simulink model "single_upsample_and_mix"  (R2022a)
settings: Solver=VariableStepAuto  StartTime=0.0  StopTime=33E-5  RelTol=1e-3
PreLoadFcn:
  | Fpass = 0.029;  % Passband Frequency
  | Fstop = 0.06;   % Stopband Frequency
  | Apass = 0.01;   % Passband Ripple (dB)
  | Astop = 100;    % Stopband Attenuation (dB)
  | h = fdesign.interpolator(16, 'Lowpass', 'fp,fst,ap,ast', Fpass, Fstop, ...
  |     Apass, Astop);
  | Hd = design(h, 'equiripple', ...
  |     'MinOrder', 'any', ...
  |     'StopbandShape', 'flat', ...
  |     'SystemObject', true);
  | set(Hd, ...
  |     'CoefficientsDataType', 'Custom', ...
  |     'CustomCoefficientsDataType', numerictype([],27,26));
  | h324=Hd.Numerator();
InitFcn:
  | Fbits=32; %frequency resolution
  | Abits=16; %Sin/COS table depth is 2^Abits
  | Dbits=16; %Sin/COS table width is 1..-Dbits
  | 
  | 
  | clk = 500e+6; % Hz
  | sample_rate = 1/2e+9; % 2GHz
  | SSR = 4;%ceil((1/sample_rate)*(1/clk));
  | Tclk = 1/clk;
  | Ts = sample_rate;
  | 
  | Is = 125e6;
  | Tis = 1/Is;
  | 
  | % FIR filter chain variables
  | pos = 1000/16*[0:16]*1E6;
  | channels = [pos,fliplr(pos(2:16)).*-1];
  | 
  | Fpass = 0.029;  % Passband Frequency
  | Fstop = 0.06;   % Stopband Frequency
  | Apass = 0.01;   % Passband Ripple (dB)
  | Astop = 100;    % Stopband Attenuation (dB)
  | h = fdesign.interpolator(16, 'Lowpass', 'fp,fst,ap,ast', Fpass, Fstop, ...
  |     Apass, Astop);
  | Hd = design(h, 'equiripple', ...
  |     'MinOrder', 'any', ...
  |     'StopbandShape', 'flat', ...
  |     'SystemObject', true);
  | set(Hd, ...
  |     'CoefficientsDataType', 'Custom', ...
  |     'CustomCoefficientsDataType', numerictype([],27,26));
  | h324=Hd.Numerator();
StartFcn:
  | start_time = tic;
StopFcn:
  | stop_time = toc(start_time)/60
undefined symbols (not defined in the file or in its folder): S, vsva2197, xcvc1902
libraries: hdlBasic x32, hdlSSR x15, hdlDSPIP x4, hdlUtilities x2, dspsigattribs x1, dspmlti4 x1, dspsrcs4 x1, vmcUtilities x1
settings Model: Creator=admin  LastModifiedBy=amd
settings SolverCC: AlgebraicLoopSolver=TrustRegion
settings DataIOCC: ReturnWorkspaceOutputs=off
settings DebuggingCC: UnconnectedInputMsg=warning  UnconnectedOutputMsg=warning  UnconnectedLineMsg=warning  SFMachineParentedDataDiag=warning  ArithmeticOperatorsInVariantConditions=warning
settings SFSimCC: SimUseLocalCustomCode=off  CustomCodeUndefinedFunction=UseInterfaceOnly
settings RTWCC: RTWUseLocalCustomCode=off  DLArmComputeVersion=19.05
settings CodeAppCC: StateflowObjectComments=on

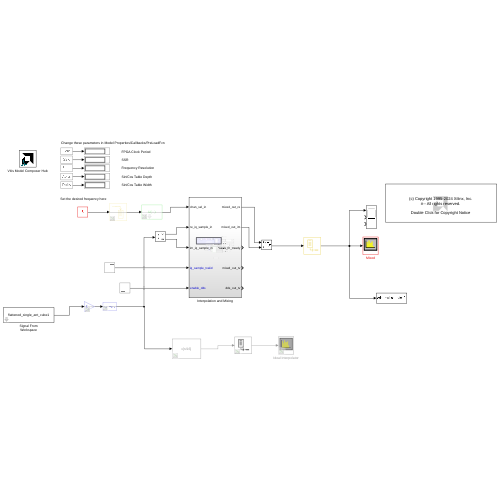
[thumbnail: Simulink's stored preview of the top-level diagram]
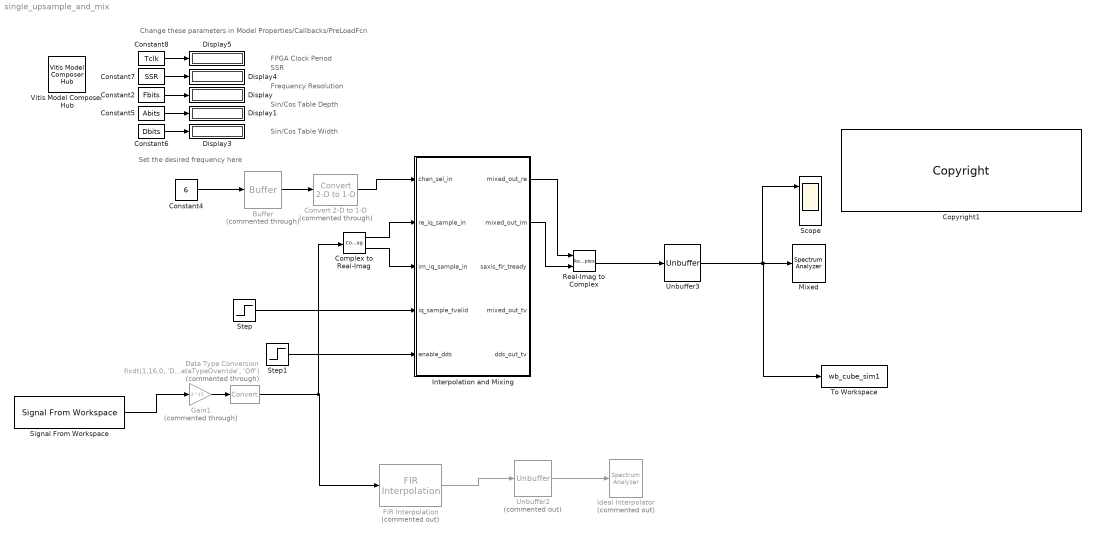
== system single_upsample_and_mix ==
  note: Frequency Resolution
  note: Set the desired frequency here
  note: Change these parameters in Model Properties/Callbacks/PreLoadFcn
  note: SSR
  note: FPGA Clock Period
  note: Sin/Cos Table Width
  note: Sin/Cos Table Depth
  Buffer : Buffer  Commented=through  N=SSR  OutputFrames=off
  Complex to Real-Imag : ComplexToRealImag
  Constant2 : Constant  Value=Fbits  OutDataTypeStr=int32  SampleTime=-1
  Constant4 : Constant  Value=6  OutDataTypeStr=fixdt(0,5,0)  SampleTime=-1
  Constant5 : Constant  Value=Abits  OutDataTypeStr=int32  SampleTime=-1
  Constant6 : Constant  Value=Dbits  OutDataTypeStr=int32  SampleTime=-1
  Constant7 : Constant  Value=SSR  OutDataTypeStr=int32  SampleTime=-1
  Constant8 : Constant  Value=Tclk  OutDataTypeStr=double  SampleTime=-1
  Convert 2-D to 1-D : dspsigattribs/Convert 2-D to 1-D  Commented=through
      settings: SourceProductBaseCode=DS
  Copyright1 : hdlUtilities/Copyright  copyrighttext="Copyright (c) 2024  by  Xilinx, Inc. All rights reserved.<br><br>This file contains proprietary, confidential information of Xilinx, Inc., is distributed under license from Xilinx, Inc., and may be used, copied and/or disclosed only pursuant to the terms of a valid license agreement with Xilinx, Inc. Xilinx hereby grants you a license to use this file solely for design, simulation, implementation and creation of design files limited to Xilinx devices or technologies. Use with non-Xilinx devices or technologies is expressly prohibited and immediately terminates your license unless covered by a separate agreement.<br><br>Xilinx is providing this design, code, or information \"as-is\" solely for use in developing programs and solutions for Xilinx devices, with no obligation on the part of Xilinx to provide support. By providing this design, code, or information as one possible implementation of this feature, application or standard, Xilinx is making no representation that this implementation is free from any claims of infringement. You are responsible for obtaining any rights you may require for your implementation. Xilinx expressly disclaims any warranty whatsoever with respect to the adequacy of the implementation, including but not limited to any warranties or representations that this implementation is free from claims of infringement, implied warranties of merchantability or fitness for a particular purpose.<br><br>Xilinx products are not intended for use in life support appliances, devices, or systems. Use in such applications is expressly prohibited.<br><br>Any modifications that are made to the Source Code are done at the user's sole risk and will be unsupported.<br><br>This copyright and support notice must be retained as part of this text at all times. (c) Copyright 1995-2024 Xilinx, Inc. All rights reserved."  block_type=copyright
  Data Type Conversion : DataTypeConversion  Commented=through  OutDataTypeStr=fixdt(1,16,0, 'DataTypeOverride', 'Off')  SaturateOnIntegerOverflow=off  RndMeth=Floor  LockScale=on
  Display{,1,3..5} (5 alike) : Display
  FIR Interpolation : dspmlti4/FIR Interpolation  Commented=on  FilterSource=Dialog parameters  PrivateCoeffs=0  h=h512  L=16  FilterObject=FINTERP  InputProcessing=Columns as channels (frame based)  framing=Enforce single-rate processing  outputBufInitCond=0  roundingMode=Floor  overflowMode=off  firstCoeffDataTypeStr=Inherit: Same word length as input  firstCoeffMin=[]  firstCoeffMax=[]  firstCoeffLastDataTypeStr=Inherit: Same word length as input  outputDataTypeStr=Inherit: Same as accumulator  outputMin=[]  outputMax=[]  outputLastDataTypeStr=Inherit: Same as accumulator
  Gain1 : Gain  Commented=through  Gain=2^15
  Ideal Interpolator : SpectrumAnalyzer  Commented=on
  Interpolation and Mixing : Subsystem
  Mixed : SpectrumAnalyzer
  Real-Imag to Complex : RealImagToComplex
  Scope : Scope  NumInputPorts=3
  Signal From Workspace : dspsrcs4/Signal From Workspace  X=flattened_single_ant_cube1  Ts=Tis  nsamps=1  OutputAfterFinalValue=Cyclic repetition  ignoreOrWarnInputAndFrameLengths=off  OutputFrames=off
  Step : Step  Time=Tis  OutDataTypeStr=Inherit: Inherit via back propagation  SampleTime=0
  Step1 : Step  Time=Tis  OutDataTypeStr=Inherit: Inherit via back propagation  SampleTime=0
  To Workspace : ToWorkspace  VariableName=wb_cube_sim1  SaveFormat=Timeseries  SampleTime=-1
  Unbuffer2 : Unbuffer  Commented=on
  Unbuffer3 : Unbuffer
  Vitis Model Composer Hub : vmcUtilities/Vitis Model Composer Hub  Tag=genX  CodeGeneration=off  TargetDirectory=./code  ExportType=System Generator  IpVendor=xilinx.com  IpLibrary=hls  IpVersion=1.0  IpHWLanguage=Verilog  AieCompilerOptions={}  AieSimulatorOptions={}  CreateTestbench=off  TestbenchStackSize=10  RunRtlSim=off  RunCSim=off  RunAieSim=off  AieSimTimeout=50000  RunAieSimProfiling=off  LaunchVitisAnalyzer=off  PlotOutput=off  RunX86Sim=off  X86SimTimeout=10  GenHwImage=off  GenLibadfXo=off  PlatformType=Not Specified  HwSystemType=Baremetal  HwValidationTarget=hw  ProjDevice=Versal VCK190 Evaluation Platform (xcvc1902-vsva2197-2MP-e-S)  ProjDevicePart=xcvc1902-vsva2197-2MP-e-S  AIEType=AIE  SamplePeriod=-1  ClockFrequency=200  DataPathParallelism=1  xilinxfamily=versalaicore  part=xcvc1902  speed=-2MP-e-S  package=vsva2197  directory=C:/work/tmp/v7_rc2  testbench=off  incr_netlist=off  synthesis_tool=Vivado  clock_wrapper=Clock Enables  dbl_ovrd=According to Block Masks  dcm_input_clock_period=10  sysclk_period=(1e+9)/clk  simulink_period=1/clk  eval_field=0  IPInfoJsonString="{\"HDLSubsystem\":{\"SubsystemName\":\"Interpolation and Mixing\",\"IPName\":\"stap_upsampler\",\"IPLibrary\":\"VMC\",\"IPVendor\":\"User Company\",\"IPVersion\":\"1.0\"}}"  LogFileName=''  NThreads=4
  wires:
  Constant4/1 -> Buffer/1
  Buffer/1 -> Convert 2-D to 1-D/1
  Constant2/1 -> Display/1
  Constant6/1 -> Display3/1
  Constant7/1 -> Display4/1
  Constant8/1 -> Display5/1
  Unbuffer3/1 -> To Workspace/1, Mixed/1, Scope/1
  Constant5/1 -> Display1/1
  Convert 2-D to 1-D/1 -> Interpolation and Mixing/1(chan_sel_in)
  FIR Interpolation/1 -> Unbuffer2/1
  Unbuffer2/1 -> Ideal Interpolator/1
  Gain1/1 -> Data Type Conversion/1
  Signal From Workspace/1 -> Gain1/1
  Data Type Conversion/1 -> Complex to Real-Imag/1, FIR Interpolation/1
  Interpolation and Mixing/2(mixed_out_im) -> Real-Imag to Complex/2
  Interpolation and Mixing/1(mixed_out_re) -> Real-Imag to Complex/1
  Real-Imag to Complex/1 -> Unbuffer3/1
  Complex to Real-Imag/1 -> Interpolation and Mixing/2(re_iq_sample_in)
  Complex to Real-Imag/2 -> Interpolation and Mixing/3(im_iq_sample_in)
  Step/1 -> Interpolation and Mixing/4(iq_sample_tvalid)
  Step1/1 -> Interpolation and Mixing/5(enable_dds)

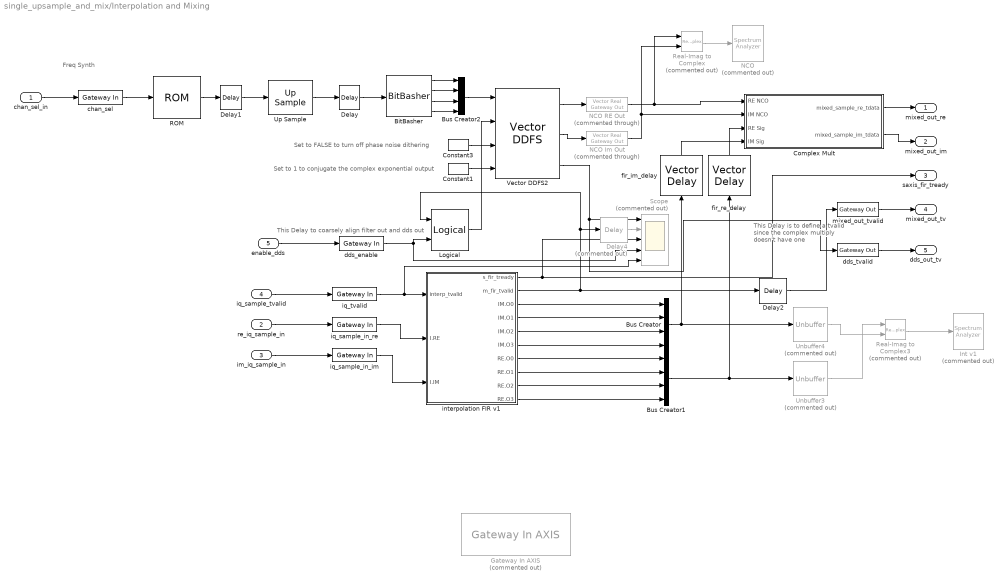
== system single_upsample_and_mix/Interpolation and Mixing ==
  note: Freq Synth
  note: Set to 1 to conjugate the complex exponential output
  note: Set to FALSE to turn off phase noise dithering
  note: This Delay to coarsely align filter out and dds out
  note: This Delay is to define a tvalid since
      | the complex multiply doesn't have one
  chan_sel_in : Inport  SampleTime=Tis
  re_iq_sample_in : Inport  Port=2
  im_iq_sample_in : Inport  Port=3
  iq_sample_tvalid : Inport  Port=4  SampleTime=Tis
  enable_dds : Inport  Port=5  SampleTime=Tclk
  BitBasher : hdlBasic/BitBasher  bitexpr=|  display_expr=off  sr_1=a  arith_type1="Signed  (2's comp)"  bin_pt1=0  sr_2=b  arith_type2="Signed  (2's comp)"  bin_pt2=0  sr_3=c  arith_type3="Signed  (2's comp)"  bin_pt3=0  sr_4=d  arith_type4="Signed  (2's comp)"  bin_pt4=0  XmcBlockStatus=1  maskContainerNames=group1  block_type=bitbasher  block_config=sysgen:BitBasher_config
      | a={e}
      | b={e}
      | c={e}
      | d={e}
  Bus Creator : BusCreator  Inputs=4
  Bus Creator1 : BusCreator  Inputs=4
  Bus Creator2 : BusCreator  Inputs=4
  Complex Mult : Subsystem
  Constant1 : hdlBasic/Constant  const=1  gui_display_data_type=Fixed-point  arith_type=Unsigned  n_bits=1  bin_pt=0  preci_type=Single  exp_width=8  frac_width=24  explicit_period=on  period=Tclk  XmcBlockStatus=1  maskContainerNames=tabcontainer1  block_type=constant  block_config=sysgen:Constant_config
  Constant3 : hdlBasic/Constant  const=1  gui_display_data_type=Boolean  arith_type=Boolean  n_bits=1  bin_pt=0  preci_type=Single  exp_width=8  frac_width=24  explicit_period=on  period=Tclk  XmcBlockStatus=1  maskContainerNames=tabcontainer1  block_type=constant  block_config=sysgen:Constant_config
  Delay : hdlBasic/Delay  rst=off  en=off  latency=1  reg_retiming=off  XmcBlockStatus=1  maskContainerNames=group1  block_type=delay  block_config=sysgen:Delay_config
  Delay1 : hdlBasic/Delay  rst=off  en=off  latency=1  reg_retiming=off  XmcBlockStatus=1  maskContainerNames=group1  block_type=delay  block_config=sysgen:Delay_config
  Delay2 : hdlBasic/Delay  rst=off  en=off  latency=5  reg_retiming=off  XmcBlockStatus=1  maskContainerNames=group1  block_type=delay  block_config=sysgen:Delay_config
  Delay4 : hdlBasic/Delay  Commented=on  rst=off  en=off  latency=13  reg_retiming=off  XmcBlockStatus=1  maskContainerNames=group1  block_type=delay  block_config=sysgen:Delay_config
  Gateway In AXIS : hdlUtilities/Gateway In AXIS  Commented=on  gui_display_data_type=Fixed-point  arith_type=Signed (2's comp)  n_bits=1  bin_pt=0  preci_type=Custom  exp_width=16  frac_width=24  quantization=Truncate  overflow=Flag as error  OutSampleTime=1  block_type=gatewayinaxi  XmcBlockStatus=1
  Int v1 : SpectrumAnalyzer  Commented=on
  Logical : hdlBasic/Logical  logical_function=OR  inputs=2  en=off  latency=1  precision=User Defined  arith_type=Boolean  n_bits=1  bin_pt=0  align_bp=on  overflow=[]  quantization=[]  XmcBlockStatus=1  maskContainerNames=tabcontainer1  block_type=logical  block_config=sysgen:Logical_config
  NCO : SpectrumAnalyzer  Commented=on
  NCO Im Out : hdlSSR/Vector Real Gateway Out  Commented=through  inherit_from_input=off  hdl_port=off  sg_ssr=4  rows=1  columns=1  UseAsDAC=off  DACChannel='1'  interface=None  automatic_assignment=on  address_offset=hex2dec('00')  intf_name=''  intf_description=''  timing_constraint=None  locs_specified=off  LOCs={}  io_standard={}  block_type=realgatewayout_ssr  XmcBlockStatus=1  sg_ssr_prev=4  maskContainerNames=group4  block_width_w=590  block_height_w=620  block_width=620  block_height=750
  NCO RE Out : hdlSSR/Vector Real Gateway Out  Commented=through  inherit_from_input=off  hdl_port=off  sg_ssr=4  rows=1  columns=1  UseAsDAC=off  DACChannel='1'  interface=None  automatic_assignment=on  address_offset=hex2dec('00')  intf_name=''  intf_description=''  timing_constraint=None  locs_specified=off  LOCs={}  io_standard={}  block_type=realgatewayout_ssr  XmcBlockStatus=1  sg_ssr_prev=4  maskContainerNames=group4  block_width_w=590  block_height_w=620  block_width=620  block_height=750
  ROM : hdlBasic/ROM  depth=32  initVector=channels*Ts*2^Fbits  distributed_mem=Distributed memory  rst=off  init_reg=0  en=off  latency=1  gui_display_data_type=Fixed-point  arith_type="Signed  (2's comp)"  n_bits=32  bin_pt=0  preci_type=Single  exp_width=8  frac_width=24  optimize=Area  use_rpm=on  simulation_type=fast_sim  XmcBlockStatus=1  maskContainerNames=tabcontainer1  block_type=sprom  block_config=sysgen:SPROM_config
  Real-Imag to Complex : RealImagToComplex  Commented=on
  Real-Imag to Complex3 : RealImagToComplex  Commented=on
  Scope : Scope  Commented=on  NumInputPorts=5
  Unbuffer3 : Unbuffer  Commented=on
  Unbuffer4 : Unbuffer  Commented=on
  Up Sample : hdlBasic/Up Sample  sample_ratio=4  copy_samples=on  en=off  latency=1  XmcBlockStatus=1  maskContainerNames=group1  block_type=usamp  block_config=sysgen:Upsample_config
  Vector DDFS2 : hdlSSR/Vector DDFS  sg_ssr=SSR  Fbits=Fbits  Abits=Abits  Dbits=Dbits  block_type=ddfs_ssr  XmcBlockStatus=1  sg_ssr_prev=4  maskContainerNames=group1
      settings: SourceProductName=Xilinx SSR Blockset
  chan_sel : hdlBasic/Gateway In  gui_display_data_type=Fixed-point  arith_type=Unsigned  n_bits=5  bin_pt=0  preci_type=Single  exp_width=8  frac_width=24  rows=1  columns=1  quantization=Truncate  overflow=Wrap  period=Tis  UseAsADC=off  ADCChannel='1'  interface=None  automatic_assignment=on  address_offset=hex2dec('00')  intf_name='channel_sel'  intf_description='0:31 mix channel select'  default_value=0  timing_constraint=None  locs_specified=off  LOCs={}  io_standard={}  inherit_from_input=off  hdl_port=on  XmcBlockStatus=1  maskContainerNames=group4  block_type=gatewayin  block_config=sysgen:gateway_in_config  block_width_w=590  block_height_w=620  block_width=640  block_height=850
  dds_enable : hdlBasic/Gateway In  gui_display_data_type=Boolean  arith_type=Boolean  n_bits=16  bin_pt=14  preci_type=Single  exp_width=8  frac_width=24  rows=1  columns=1  quantization="Round  (unbiased: +/- Inf)"  overflow=Saturate  period=Tclk  UseAsADC=off  ADCChannel='1'  interface=None  automatic_assignment=on  address_offset=hex2dec('00')  intf_name=''  intf_description=''  default_value=0  timing_constraint=None  locs_specified=off  LOCs={}  io_standard={}  inherit_from_input=off  hdl_port=on  XmcBlockStatus=1  maskContainerNames=group4  block_type=gatewayin  block_config=sysgen:gateway_in_config  block_width_w=590  block_height_w=620  block_width=640  block_height=850
  dds_tvalid : hdlBasic/Gateway Out  inherit_from_input=on  hdl_port=on  rows=1  columns=1  UseAsDAC=off  DACChannel='1'  interface=None  automatic_assignment=on  address_offset=hex2dec('00')  intf_name=''  intf_description=''  timing_constraint=None  locs_specified=off  LOCs={}  io_standard={}  XmcBlockStatus=1  maskContainerNames=group4  block_type=gatewayout  block_config=sysgen:gateway_out_config  block_width_w=590  block_height_w=620  block_width=620  block_height=750
  fir_im_delay : hdlSSR/Vector Delay  rst=off  en=off  vectorize_en=off  sg_latency=1  sg_ssr=4  reg_retiming=off  block_type=delay_ssr  XmcBlockStatus=1  sg_ssr_prev=4  maskContainerNames=group1
  fir_re_delay : hdlSSR/Vector Delay  rst=off  en=off  vectorize_en=off  sg_latency=1  sg_ssr=4  reg_retiming=off  block_type=delay_ssr  XmcBlockStatus=1  sg_ssr_prev=4  maskContainerNames=group1
  interpolation FIR v1 : Subsystem
  iq_sample_in_im : hdlBasic/Gateway In  gui_display_data_type=Fixed-point  arith_type=Signed (2's comp)  n_bits=16  bin_pt=15  preci_type=Single  exp_width=8  frac_width=24  rows=1  columns=1  quantization=Truncate  overflow=Saturate  period=Tis  UseAsADC=off  ADCChannel='1'  interface=None  automatic_assignment=on  address_offset=hex2dec('00')  intf_name=''  intf_description=''  default_value=0  timing_constraint=None  locs_specified=off  LOCs={}  io_standard={}  inherit_from_input=off  hdl_port=on  XmcBlockStatus=1  maskContainerNames=group4  block_type=gatewayin  block_config=sysgen:gateway_in_config  block_width_w=590  block_height_w=620  block_width=640  block_height=850
  iq_sample_in_re : hdlBasic/Gateway In  gui_display_data_type=Fixed-point  arith_type=Signed (2's comp)  n_bits=16  bin_pt=15  preci_type=Single  exp_width=8  frac_width=24  rows=1  columns=1  quantization=Truncate  overflow=Saturate  period=Tis  UseAsADC=off  ADCChannel='1'  interface=None  automatic_assignment=on  address_offset=hex2dec('00')  intf_name=''  intf_description=''  default_value=0  timing_constraint=None  locs_specified=off  LOCs={}  io_standard={}  inherit_from_input=off  hdl_port=on  XmcBlockStatus=1  maskContainerNames=group4  block_type=gatewayin  block_config=sysgen:gateway_in_config  block_width_w=590  block_height_w=620  block_width=640  block_height=850
  iq_tvalid : hdlBasic/Gateway In  gui_display_data_type=Boolean  arith_type=Boolean  n_bits=16  bin_pt=14  preci_type=Single  exp_width=8  frac_width=24  rows=1  columns=1  quantization="Round  (unbiased: +/- Inf)"  overflow=Saturate  period=Tis  UseAsADC=off  ADCChannel='1'  interface=None  automatic_assignment=on  address_offset=hex2dec('00')  intf_name=''  intf_description=''  default_value=0  timing_constraint=None  locs_specified=off  LOCs={}  io_standard={}  inherit_from_input=off  hdl_port=on  XmcBlockStatus=1  maskContainerNames=group4  block_type=gatewayin  block_config=sysgen:gateway_in_config  block_width_w=590  block_height_w=620  block_width=640  block_height=850
  mixed_out_tvalid : hdlBasic/Gateway Out  inherit_from_input=on  hdl_port=on  rows=1  columns=1  UseAsDAC=off  DACChannel='1'  interface=None  automatic_assignment=on  address_offset=hex2dec('00')  intf_name=''  intf_description=''  timing_constraint=None  locs_specified=off  LOCs={}  io_standard={}  XmcBlockStatus=1  maskContainerNames=group4  block_type=gatewayout  block_config=sysgen:gateway_out_config  block_width_w=590  block_height_w=620  block_width=620  block_height=750
  mixed_out_re : Outport  SampleTime=Tclk
  mixed_out_im : Outport  Port=2  SampleTime=Tclk
  saxis_fir_tready : Outport  Port=3  SampleTime=Tclk
  mixed_out_tv : Outport  Port=4  SampleTime=Tclk
  dds_out_tv : Outport  Port=5  SampleTime=Tclk
  wires:
  BitBasher/1 -> Bus Creator2/1
  iq_sample_tvalid/1 -> iq_tvalid/1
  iq_tvalid/1 -> Scope/5, interpolation FIR v1/1("interp_tvalid ")
  iq_sample_in_im/1 -> interpolation FIR v1/3("I.IM ")
  NCO RE Out/1 -> Real-Imag to Complex/1, Complex Mult/1(RE NCO)
  chan_sel/1 -> ROM/1
  Complex Mult/2(mixed_sample_im_tdata) -> mixed_out_im/1
  interpolation FIR v1/6(IM.O3) -> Bus Creator/4
  im_iq_sample_in/1 -> iq_sample_in_im/1
  Constant1/1 -> Vector DDFS2/4
  Delay1/1 -> Up Sample/1
  Real-Imag to Complex/1 -> NCO/1
  Unbuffer3/1 -> Real-Imag to Complex3/1
  iq_sample_in_re/1 -> interpolation FIR v1/2("I.RE ")
  Delay/1 -> BitBasher/1
  re_iq_sample_in/1 -> iq_sample_in_re/1
  Up Sample/1 -> Delay/1
  Real-Imag to Complex3/1 -> Int v1/1
  Unbuffer4/1 -> Real-Imag to Complex3/2
  interpolation FIR v1/7(RE.O0) -> Bus Creator1/1
  interpolation FIR v1/10(RE.O3) -> Bus Creator1/4
  interpolation FIR v1/9(RE.O2) -> Bus Creator1/3
  interpolation FIR v1/8(RE.O1) -> Bus Creator1/2
  interpolation FIR v1/5(IM.O2) -> Bus Creator/3
  interpolation FIR v1/4(IM.O1) -> Bus Creator/2
  interpolation FIR v1/3(IM.O0) -> Bus Creator/1
  Complex Mult/1(mixed_sample_re_tdata) -> mixed_out_re/1
  Bus Creator/1 -> fir_im_delay/1, Unbuffer4/1
  Bus Creator1/1 -> Unbuffer3/1, fir_re_delay/1
  ROM/1 -> Delay1/1
  BitBasher/4 -> Bus Creator2/4
  BitBasher/3 -> Bus Creator2/3
  NCO Im Out/1 -> Complex Mult/2(IM NCO), Real-Imag to Complex/2
  BitBasher/2 -> Bus Creator2/2
  Vector DDFS2/1 -> NCO RE Out/1
  Bus Creator2/1 -> Vector DDFS2/1
  Vector DDFS2/2 -> NCO Im Out/1
  Constant3/1 -> Vector DDFS2/3
  chan_sel_in/1 -> chan_sel/1
  interpolation FIR v1/2(" m_fir_tvalid") -> Delay4/1, Logical/1, Delay2/1
  Vector DDFS2/3 -> dds_tvalid/1, Scope/1
  interpolation FIR v1/1(" s_fir_tready") -> saxis_fir_tready/1, Scope/3
  dds_enable/1 -> Logical/2, Scope/4
  enable_dds/1 -> dds_enable/1
  mixed_out_tvalid/1 -> mixed_out_tv/1
  Delay2/1 -> mixed_out_tvalid/1
  dds_tvalid/1 -> dds_out_tv/1
  Delay4/1 -> Scope/2
  fir_re_delay/1 -> Complex Mult/3(RE Sig)
  fir_im_delay/1 -> Complex Mult/4(IM Sig)
  Logical/1 -> Vector DDFS2/2

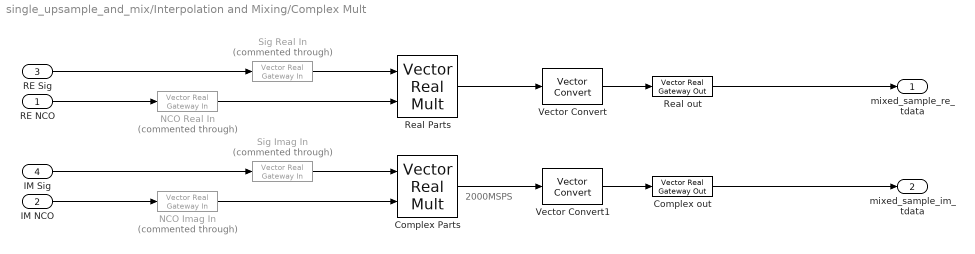
== system single_upsample_and_mix/Interpolation and Mixing/Complex Mult ==
  note: 2000MSPS
  RE NCO : Inport  SampleTime=Tclk
  IM NCO : Inport  Port=2  SampleTime=Tclk
  RE Sig : Inport  Port=3  SampleTime=Tclk
  IM Sig : Inport  Port=4  SampleTime=Tclk
  Complex Parts : hdlSSR/Vector Real Mult  precision=Full  arith_type="Signed  (2's comp)"  n_bits=16  bin_pt=15  quantization="Round  (unbiased: +/- Inf)"  overflow=Flag as error  en=off  sg_latency=3  sg_ssr=SSR  use_behavioral_HDL=off  opt=Speed  use_embedded=on  optimum_pipeline=off  pipeline=on  use_rpm=on  placement_style=Triangular  block_type=realmult_ssr  XmcBlockStatus=1  sg_ssr_prev=4  maskContainerNames=group1
      settings: SourceProductName=Xilinx SSR Blockset
  Complex out : hdlSSR/Vector Real Gateway Out  inherit_from_input=on  hdl_port=on  sg_ssr=SSR  rows=1  columns=1  UseAsDAC=off  DACChannel='1'  interface=None  automatic_assignment=on  address_offset=hex2dec('00')  intf_name=''  intf_description=''  timing_constraint=None  locs_specified=off  LOCs={}  io_standard={}  block_type=realgatewayout_ssr  XmcBlockStatus=1  sg_ssr_prev=4  maskContainerNames=group4  block_width_w=590  block_height_w=620  block_width=620  block_height=750
      settings: SourceProductName=Xilinx SSR Blockset
  NCO Imag In : hdlSSR/Vector Real Gateway In  Commented=through  gui_display_data_type=Fixed-point  arith_type=Signed (2's comp)  n_bits=18  bin_pt=16  preci_type=Single  exp_width=8  frac_width=24  quantization="Round  (unbiased: +/- Inf)"  overflow=Saturate  period=Tclk  sg_ssr=4  UseAsADC=off  ADCChannel='1'  interface=None  automatic_assignment=on  address_offset=hex2dec('00')  intf_name=''  intf_description=''  default_value=0  timing_constraint=None  locs_specified=off  LOCs={}  io_standard={}  inherit_from_input=off  hdl_port=on  interface_prev=1  block_type=realgatewayin_ssr  XmcBlockStatus=1  sg_ssr_prev=4  maskContainerNames=group4  block_width_w=590  block_height_w=670  block_width=640  block_height=850
  NCO Real In : hdlSSR/Vector Real Gateway In  Commented=through  gui_display_data_type=Fixed-point  arith_type=Signed (2's comp)  n_bits=18  bin_pt=16  preci_type=Single  exp_width=8  frac_width=24  quantization="Round  (unbiased: +/- Inf)"  overflow=Saturate  period=Tclk  sg_ssr=4  UseAsADC=off  ADCChannel='1'  interface=None  automatic_assignment=on  address_offset=hex2dec('00')  intf_name=''  intf_description=''  default_value=0  timing_constraint=None  locs_specified=off  LOCs={}  io_standard={}  inherit_from_input=off  hdl_port=on  interface_prev=1  block_type=realgatewayin_ssr  XmcBlockStatus=1  sg_ssr_prev=4  maskContainerNames=group4  block_width_w=590  block_height_w=670  block_width=640  block_height=850
  Real Parts : hdlSSR/Vector Real Mult  precision=Full  arith_type="Signed  (2's comp)"  n_bits=16  bin_pt=15  quantization="Round  (unbiased: +/- Inf)"  overflow=Flag as error  en=off  sg_latency=3  sg_ssr=SSR  use_behavioral_HDL=off  opt=Speed  use_embedded=on  optimum_pipeline=off  pipeline=on  use_rpm=on  placement_style=Triangular  block_type=realmult_ssr  XmcBlockStatus=1  sg_ssr_prev=4  maskContainerNames=group1
      settings: SourceProductName=Xilinx SSR Blockset
  Real out : hdlSSR/Vector Real Gateway Out  inherit_from_input=on  hdl_port=on  sg_ssr=SSR  rows=1  columns=1  UseAsDAC=off  DACChannel='1'  interface=None  automatic_assignment=on  address_offset=hex2dec('00')  intf_name=''  intf_description=''  timing_constraint=None  locs_specified=off  LOCs={}  io_standard={}  block_type=realgatewayout_ssr  XmcBlockStatus=1  sg_ssr_prev=4  maskContainerNames=group4  block_width_w=590  block_height_w=620  block_width=620  block_height=750
      settings: SourceProductName=Xilinx SSR Blockset
  Sig Imag In : hdlSSR/Vector Real Gateway In  Commented=through  gui_display_data_type=Fixed-point  arith_type=Signed (2's comp)  n_bits=27  bin_pt=26  preci_type=Single  exp_width=8  frac_width=24  quantization="Round  (unbiased: +/- Inf)"  overflow=Saturate  period=Tclk  sg_ssr=4  UseAsADC=off  ADCChannel='1'  interface=None  automatic_assignment=on  address_offset=hex2dec('00')  intf_name=''  intf_description=''  default_value=0  timing_constraint=None  locs_specified=off  LOCs={}  io_standard={}  inherit_from_input=off  hdl_port=on  interface_prev=1  block_type=realgatewayin_ssr  XmcBlockStatus=1  sg_ssr_prev=4  maskContainerNames=group4  block_width_w=590  block_height_w=670  block_width=640  block_height=850
  Sig Real In : hdlSSR/Vector Real Gateway In  Commented=through  gui_display_data_type=Fixed-point  arith_type=Signed (2's comp)  n_bits=27  bin_pt=26  preci_type=Single  exp_width=8  frac_width=24  quantization="Round  (unbiased: +/- Inf)"  overflow=Saturate  period=Tclk  sg_ssr=4  UseAsADC=off  ADCChannel='1'  interface=None  automatic_assignment=on  address_offset=hex2dec('00')  intf_name=''  intf_description=''  default_value=0  timing_constraint=None  locs_specified=off  LOCs={}  io_standard={}  inherit_from_input=off  hdl_port=on  interface_prev=1  block_type=realgatewayin_ssr  XmcBlockStatus=1  sg_ssr_prev=4  maskContainerNames=group4  block_width_w=590  block_height_w=670  block_width=640  block_height=850
  Vector Convert : hdlSSR/Vector Convert  gui_display_data_type=Fixed-point  arith_type=Signed (2's comp)  n_bits=16  bin_pt=15  float_type=Single  exp_bits=8  fraction_bits=24  quantization="Round  (unbiased: +/- Inf)"  overflow=Saturate  en=off  sg_latency=1  sg_ssr=4  pipeline=off  block_type=convert_ssr  XmcBlockStatus=1  sg_ssr_prev=4  maskContainerNames=group2
  Vector Convert1 : hdlSSR/Vector Convert  gui_display_data_type=Fixed-point  arith_type=Signed (2's comp)  n_bits=16  bin_pt=15  float_type=Single  exp_bits=8  fraction_bits=24  quantization="Round  (unbiased: +/- Inf)"  overflow=Saturate  en=off  sg_latency=1  sg_ssr=4  pipeline=off  block_type=convert_ssr  XmcBlockStatus=1  sg_ssr_prev=4  maskContainerNames=group2
  mixed_sample_re_tdata : Outport  SampleTime=Tclk
  mixed_sample_im_tdata : Outport  Port=2  SampleTime=Tclk
  wires:
  Real Parts/1 -> Vector Convert/1
  RE Sig/1 -> Sig Real In/1
  RE NCO/1 -> NCO Real In/1
  Complex Parts/1 -> Vector Convert1/1
  IM NCO/1 -> NCO Imag In/1
  Vector Convert/1 -> Real out/1
  IM Sig/1 -> Sig Imag In/1
  Vector Convert1/1 -> Complex out/1
  Complex out/1 -> mixed_sample_im_tdata/1
  Sig Real In/1 -> Real Parts/1
  Sig Imag In/1 -> Complex Parts/1
  NCO Real In/1 -> Real Parts/2
  NCO Imag In/1 -> Complex Parts/2
  Real out/1 -> mixed_sample_re_tdata/1

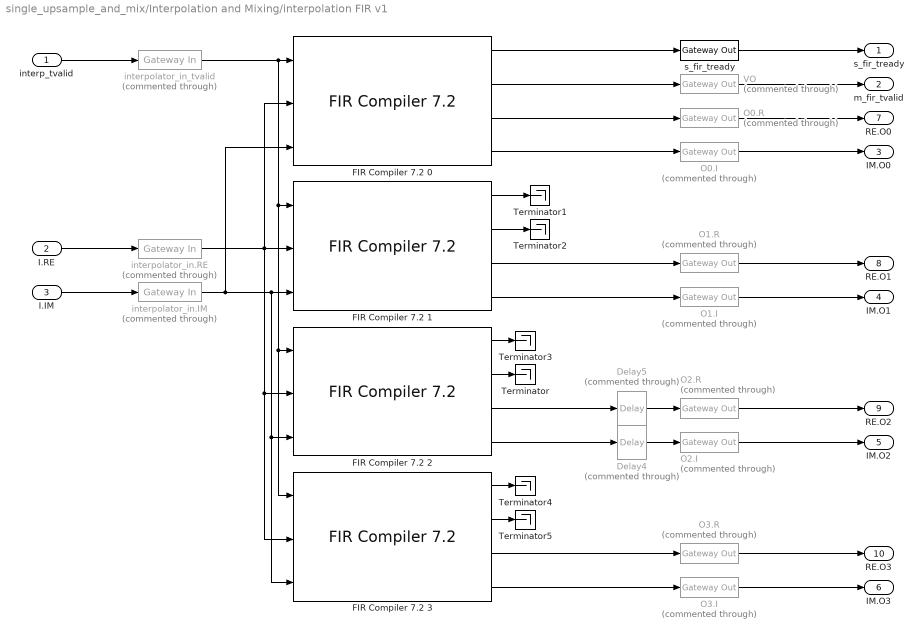
== system single_upsample_and_mix/Interpolation and Mixing/interpolation FIR v1 ==
  "interp_tvalid " : Inport  SampleTime=Tis
  "I.RE " : Inport  Port=2
  "I.IM " : Inport  Port=3
  Delay4 : hdlBasic/Delay  Commented=through  rst=off  en=off  latency=8  reg_retiming=off  XmcBlockStatus=1  maskContainerNames=group1  block_type=delay  block_config=sysgen:Delay_config
  Delay5 : hdlBasic/Delay  Commented=through  rst=off  en=off  latency=8  reg_retiming=off  XmcBlockStatus=1  maskContainerNames=group1  block_type=delay  block_config=sysgen:Delay_config
  FIR Compiler 7.2 0 : hdlDSPIP/FIR Compiler 7.2   coefficientvector=h324(1:4:end)  coefficient_sets=1  coefficient_reload=off  filter_type=Interpolation  rate_change_type=Integer  interpolation_rate=4  decimation_rate=1  zero_pack_factor=1  channel_sequence=Basic  number_channels=1  pattern_list='P4-0,P4-1,P4-2,P4-3,P4-4'  number_paths=2  ratespecification=Input_Sample_Period  sampleperiod=4  hardwareoversamplingrate=1  coefficient_sign=Signed  quantization=Quantize_Only  coefficient_width=27  bestprecision=off  coefficient_fractional_bits=26  coefficient_structure=Inferred  output_rounding_mode=Non_Symmetric_Rounding_Down  output_width=27  filter_architecture=Systolic_Multiply_Accumulate  optimization_goal=Area  optimization_list='None'  data_buffer_type=Automatic  coefficient_buffer_type=Automatic  input_buffer_type=Automatic  output_buffer_type=Automatic  preference_for_other_storage=Automatic  multi_column_support=Automatic  columnconfig='3'  inter_column_pipe_length=4  data_has_tlast=Not_Required  m_data_has_tready=off  s_data_has_fifo=off  s_data_has_tuser=Not_Required  m_data_has_tuser=Not_Required  s_config_sync_mode=On_Vector  s_config_method=Single  num_reload_slots=1  has_aclken=off  has_aresetn=off  reset_data_vector=on  trim_axipin_name=on  simulation_type=hybrid_sim  simulation_model=sysgen:xfirv7_2_cmodel  data_path_portlist={ 's_axis_data_tdata', 'm_axis_data_tdata' }  passband_min=0.0  passband_max=0.5  stopband_min=0.5  stopband_max=1.0  filter_selection=1  gui_behaviour='Sysgen_GUI'  data_sign=Signed  data_width=16  data_fractional_bits=0  data_tuser_width=1  wrapper_available=true  ip_wrap_arbitrary_binary_point=true  ip_name=FIR Compiler  ip_version=7.2  dsptool_ready=true  ipcore_usecache=true  ipcore_useipmodelcache=true  port_translation_map={ 'aclken' => 'en', 'aresetn' => 'rst' }  run_core_at_system_period=true  ipcore_xco_need_fpga_part=true  ipcore_fpga_part=[]  XmcBlockStatus=1  maskContainerNames=tabcontainer1  block_type=fir_compiler_v7_2  block_config=sysgen:rodinimport_config  block_width=820  block_height=600
  FIR Compiler 7.2 1 : hdlDSPIP/FIR Compiler 7.2   coefficientvector=h324(2:4:end)  coefficient_sets=1  coefficient_reload=off  filter_type=Interpolation  rate_change_type=Integer  interpolation_rate=4  decimation_rate=1  zero_pack_factor=1  channel_sequence=Basic  number_channels=1  pattern_list='P4-0,P4-1,P4-2,P4-3,P4-4'  number_paths=2  ratespecification=Input_Sample_Period  sampleperiod=4.000000  hardwareoversamplingrate=1  coefficient_sign=Signed  quantization=Quantize_Only  coefficient_width=27  bestprecision=off  coefficient_fractional_bits=26  coefficient_structure=Inferred  output_rounding_mode=Non_Symmetric_Rounding_Down  output_width=27  filter_architecture=Systolic_Multiply_Accumulate  optimization_goal=Area  optimization_list='None'  data_buffer_type=Automatic  coefficient_buffer_type=Automatic  input_buffer_type=Automatic  output_buffer_type=Automatic  preference_for_other_storage=Automatic  multi_column_support=Automatic  columnconfig='21'  inter_column_pipe_length=4  data_has_tlast=Not_Required  m_data_has_tready=off  s_data_has_fifo=off  s_data_has_tuser=Not_Required  m_data_has_tuser=Not_Required  s_config_sync_mode=On_Vector  s_config_method=Single  num_reload_slots=1  has_aclken=off  has_aresetn=off  reset_data_vector=on  trim_axipin_name=on  simulation_type=hybrid_sim  simulation_model=sysgen:xfirv7_2_cmodel  data_path_portlist={ 's_axis_data_tdata', 'm_axis_data_tdata' }  passband_min=0.0  passband_max=0.5  stopband_min=0.5  stopband_max=1.0  filter_selection=1  gui_behaviour='Sysgen_GUI'  data_sign=Signed  data_width=16  data_fractional_bits=0  data_tuser_width=1  wrapper_available=true  ip_wrap_arbitrary_binary_point=true  ip_name=FIR Compiler  ip_version=7.2  dsptool_ready=true  ipcore_usecache=true  ipcore_useipmodelcache=true  port_translation_map={ 'aclken' => 'en', 'aresetn' => 'rst' }  run_core_at_system_period=true  ipcore_xco_need_fpga_part=true  ipcore_fpga_part=[]  XmcBlockStatus=1  maskContainerNames=tabcontainer1  block_type=fir_compiler_v7_2  block_config=sysgen:rodinimport_config  block_width=820  block_height=600
  FIR Compiler 7.2 2 : hdlDSPIP/FIR Compiler 7.2   coefficientvector=h324(3:4:end)  coefficient_sets=1  coefficient_reload=off  filter_type=Interpolation  rate_change_type=Integer  interpolation_rate=4  decimation_rate=1  zero_pack_factor=1  channel_sequence=Basic  number_channels=1  pattern_list='P4-0,P4-1,P4-2,P4-3,P4-4'  number_paths=2  ratespecification=Input_Sample_Period  sampleperiod=4.000000  hardwareoversamplingrate=1  coefficient_sign=Signed  quantization=Quantize_Only  coefficient_width=27  bestprecision=off  coefficient_fractional_bits=26  coefficient_structure=Inferred  output_rounding_mode=Non_Symmetric_Rounding_Down  output_width=27  filter_architecture=Systolic_Multiply_Accumulate  optimization_goal=Area  optimization_list='None'  data_buffer_type=Automatic  coefficient_buffer_type=Automatic  input_buffer_type=Automatic  output_buffer_type=Automatic  preference_for_other_storage=Automatic  multi_column_support=Automatic  columnconfig='21'  inter_column_pipe_length=4  data_has_tlast=Not_Required  m_data_has_tready=off  s_data_has_fifo=off  s_data_has_tuser=Not_Required  m_data_has_tuser=Not_Required  s_config_sync_mode=On_Vector  s_config_method=Single  num_reload_slots=1  has_aclken=off  has_aresetn=off  reset_data_vector=on  trim_axipin_name=on  simulation_type=hybrid_sim  simulation_model=sysgen:xfirv7_2_cmodel  data_path_portlist={ 's_axis_data_tdata', 'm_axis_data_tdata' }  passband_min=0.0  passband_max=0.5  stopband_min=0.5  stopband_max=1.0  filter_selection=1  gui_behaviour='Sysgen_GUI'  data_sign=Signed  data_width=16  data_fractional_bits=0  data_tuser_width=1  wrapper_available=true  ip_wrap_arbitrary_binary_point=true  ip_name=FIR Compiler  ip_version=7.2  dsptool_ready=true  ipcore_usecache=true  ipcore_useipmodelcache=true  port_translation_map={ 'aclken' => 'en', 'aresetn' => 'rst' }  run_core_at_system_period=true  ipcore_xco_need_fpga_part=true  ipcore_fpga_part=[]  XmcBlockStatus=1  maskContainerNames=tabcontainer1  block_type=fir_compiler_v7_2  block_config=sysgen:rodinimport_config  block_width=820  block_height=600
  FIR Compiler 7.2 3 : hdlDSPIP/FIR Compiler 7.2   coefficientvector=h324(4:4:end)  coefficient_sets=1  coefficient_reload=off  filter_type=Interpolation  rate_change_type=Integer  interpolation_rate=4  decimation_rate=1  zero_pack_factor=1  channel_sequence=Basic  number_channels=1  pattern_list='P4-0,P4-1,P4-2,P4-3,P4-4'  number_paths=2  ratespecification=Input_Sample_Period  sampleperiod=4.000000  hardwareoversamplingrate=1  coefficient_sign=Signed  quantization=Quantize_Only  coefficient_width=27  bestprecision=off  coefficient_fractional_bits=26  coefficient_structure=Inferred  output_rounding_mode=Non_Symmetric_Rounding_Down  output_width=27  filter_architecture=Systolic_Multiply_Accumulate  optimization_goal=Area  optimization_list='None'  data_buffer_type=Automatic  coefficient_buffer_type=Automatic  input_buffer_type=Automatic  output_buffer_type=Block  preference_for_other_storage=Automatic  multi_column_support=Automatic  columnconfig='21'  inter_column_pipe_length=4  data_has_tlast=Not_Required  m_data_has_tready=off  s_data_has_fifo=off  s_data_has_tuser=Not_Required  m_data_has_tuser=Not_Required  s_config_sync_mode=On_Vector  s_config_method=Single  num_reload_slots=1  has_aclken=off  has_aresetn=off  reset_data_vector=on  trim_axipin_name=on  simulation_type=hybrid_sim  simulation_model=sysgen:xfirv7_2_cmodel  data_path_portlist={ 's_axis_data_tdata', 'm_axis_data_tdata' }  passband_min=0.0  passband_max=0.5  stopband_min=0.5  stopband_max=1.0  filter_selection=1  gui_behaviour='Sysgen_GUI'  data_sign=Signed  data_width=16  data_fractional_bits=0  data_tuser_width=1  wrapper_available=true  ip_wrap_arbitrary_binary_point=true  ip_name=FIR Compiler  ip_version=7.2  dsptool_ready=true  ipcore_usecache=true  ipcore_useipmodelcache=true  port_translation_map={ 'aclken' => 'en', 'aresetn' => 'rst' }  run_core_at_system_period=true  ipcore_xco_need_fpga_part=true  ipcore_fpga_part=[]  XmcBlockStatus=1  maskContainerNames=tabcontainer1  block_type=fir_compiler_v7_2  block_config=sysgen:rodinimport_config  block_width=820  block_height=600
  O0.I : hdlBasic/Gateway Out  Commented=through  inherit_from_input=off  hdl_port=off  rows=1  columns=1  UseAsDAC=off  DACChannel='1'  interface=None  automatic_assignment=on  address_offset=hex2dec('00')  intf_name=''  intf_description=''  timing_constraint=None  locs_specified=off  LOCs={}  io_standard={}  XmcBlockStatus=1  maskContainerNames=group4  block_type=gatewayout  block_config=sysgen:gateway_out_config  block_width_w=590  block_height_w=620  block_width=620  block_height=750
  O0.R : hdlBasic/Gateway Out  Commented=through  inherit_from_input=off  hdl_port=off  rows=1  columns=1  UseAsDAC=off  DACChannel='1'  interface=None  automatic_assignment=on  address_offset=hex2dec('00')  intf_name=''  intf_description=''  timing_constraint=None  locs_specified=off  LOCs={}  io_standard={}  XmcBlockStatus=1  maskContainerNames=group4  block_type=gatewayout  block_config=sysgen:gateway_out_config  block_width_w=590  block_height_w=620  block_width=620  block_height=750
  O1.I : hdlBasic/Gateway Out  Commented=through  inherit_from_input=off  hdl_port=off  rows=1  columns=1  UseAsDAC=off  DACChannel='1'  interface=None  automatic_assignment=on  address_offset=hex2dec('00')  intf_name=''  intf_description=''  timing_constraint=None  locs_specified=off  LOCs={}  io_standard={}  XmcBlockStatus=1  maskContainerNames=group4  block_type=gatewayout  block_config=sysgen:gateway_out_config  block_width_w=590  block_height_w=620  block_width=620  block_height=750
  O1.R : hdlBasic/Gateway Out  Commented=through  inherit_from_input=off  hdl_port=off  rows=1  columns=1  UseAsDAC=off  DACChannel='1'  interface=None  automatic_assignment=on  address_offset=hex2dec('00')  intf_name=''  intf_description=''  timing_constraint=None  locs_specified=off  LOCs={}  io_standard={}  XmcBlockStatus=1  maskContainerNames=group4  block_type=gatewayout  block_config=sysgen:gateway_out_config  block_width_w=590  block_height_w=620  block_width=620  block_height=750
  O2.I : hdlBasic/Gateway Out  Commented=through  inherit_from_input=off  hdl_port=off  rows=1  columns=1  UseAsDAC=off  DACChannel='1'  interface=None  automatic_assignment=on  address_offset=hex2dec('00')  intf_name=''  intf_description=''  timing_constraint=None  locs_specified=off  LOCs={}  io_standard={}  XmcBlockStatus=1  maskContainerNames=group4  block_type=gatewayout  block_config=sysgen:gateway_out_config  block_width_w=590  block_height_w=620  block_width=620  block_height=750
  O2.R : hdlBasic/Gateway Out  Commented=through  inherit_from_input=off  hdl_port=off  rows=1  columns=1  UseAsDAC=off  DACChannel='1'  interface=None  automatic_assignment=on  address_offset=hex2dec('00')  intf_name=''  intf_description=''  timing_constraint=None  locs_specified=off  LOCs={}  io_standard={}  XmcBlockStatus=1  maskContainerNames=group4  block_type=gatewayout  block_config=sysgen:gateway_out_config  block_width_w=590  block_height_w=620  block_width=620  block_height=750
  O3.I : hdlBasic/Gateway Out  Commented=through  inherit_from_input=off  hdl_port=off  rows=1  columns=1  UseAsDAC=off  DACChannel='1'  interface=None  automatic_assignment=on  address_offset=hex2dec('00')  intf_name=''  intf_description=''  timing_constraint=None  locs_specified=off  LOCs={}  io_standard={}  XmcBlockStatus=1  maskContainerNames=group4  block_type=gatewayout  block_config=sysgen:gateway_out_config  block_width_w=590  block_height_w=620  block_width=620  block_height=750
  O3.R : hdlBasic/Gateway Out  Commented=through  inherit_from_input=off  hdl_port=off  rows=1  columns=1  UseAsDAC=off  DACChannel='1'  interface=None  automatic_assignment=on  address_offset=hex2dec('00')  intf_name=''  intf_description=''  timing_constraint=None  locs_specified=off  LOCs={}  io_standard={}  XmcBlockStatus=1  maskContainerNames=group4  block_type=gatewayout  block_config=sysgen:gateway_out_config  block_width_w=590  block_height_w=620  block_width=620  block_height=750
  Terminator{,1..5} (6 alike) : Terminator
  VO : hdlBasic/Gateway Out  Commented=through  inherit_from_input=off  hdl_port=off  rows=1  columns=1  UseAsDAC=off  DACChannel='1'  interface=None  automatic_assignment=on  address_offset=hex2dec('00')  intf_name=''  intf_description=''  timing_constraint=None  locs_specified=off  LOCs={}  io_standard={}  XmcBlockStatus=1  maskContainerNames=group4  block_type=gatewayout  block_config=sysgen:gateway_out_config  block_width_w=590  block_height_w=620  block_width=620  block_height=750
  interpolator_in.IM : hdlBasic/Gateway In  Commented=through  gui_display_data_type=Fixed-point  arith_type=Signed (2's comp)  n_bits=16  bin_pt=15  preci_type=Single  exp_width=8  frac_width=24  rows=1  columns=1  quantization="Round  (unbiased: +/- Inf)"  overflow=Saturate  period=Tclk  UseAsADC=off  ADCChannel='1'  interface=None  automatic_assignment=on  address_offset=hex2dec('00')  intf_name=''  intf_description=''  default_value=0  timing_constraint=None  locs_specified=off  LOCs={}  io_standard={}  inherit_from_input=off  hdl_port=on  XmcBlockStatus=1  maskContainerNames=group4  block_type=gatewayin  block_config=sysgen:gateway_in_config  block_width_w=590  block_height_w=620  block_width=640  block_height=850
  interpolator_in.RE : hdlBasic/Gateway In  Commented=through  gui_display_data_type=Fixed-point  arith_type=Signed (2's comp)  n_bits=16  bin_pt=15  preci_type=Single  exp_width=8  frac_width=24  rows=1  columns=1  quantization="Round  (unbiased: +/- Inf)"  overflow=Saturate  period=Tclk  UseAsADC=off  ADCChannel='1'  interface=None  automatic_assignment=on  address_offset=hex2dec('00')  intf_name=''  intf_description=''  default_value=0  timing_constraint=None  locs_specified=off  LOCs={}  io_standard={}  inherit_from_input=off  hdl_port=on  XmcBlockStatus=1  maskContainerNames=group4  block_type=gatewayin  block_config=sysgen:gateway_in_config  block_width_w=590  block_height_w=620  block_width=640  block_height=850
  interpolator_in_tvalid : hdlBasic/Gateway In  Commented=through  gui_display_data_type=Boolean  arith_type=Boolean  n_bits=16  bin_pt=0  preci_type=Single  exp_width=8  frac_width=24  rows=1  columns=1  quantization="Round  (unbiased: +/- Inf)"  overflow=Saturate  period=Tis  UseAsADC=off  ADCChannel='1'  interface=None  automatic_assignment=on  address_offset=hex2dec('00')  intf_name=''  intf_description=''  default_value=0  timing_constraint=None  locs_specified=off  LOCs={}  io_standard={}  inherit_from_input=off  hdl_port=on  XmcBlockStatus=1  maskContainerNames=group4  block_type=gatewayin  block_config=sysgen:gateway_in_config  block_width_w=590  block_height_w=620  block_width=640  block_height=850
  s_fir_tready : hdlBasic/Gateway Out  inherit_from_input=on  hdl_port=on  rows=1  columns=1  UseAsDAC=off  DACChannel='1'  interface=None  automatic_assignment=on  address_offset=hex2dec('00')  intf_name=''  intf_description=''  timing_constraint=None  locs_specified=off  LOCs={}  io_standard={}  XmcBlockStatus=1  maskContainerNames=group4  block_type=gatewayout  block_config=sysgen:gateway_out_config  block_width_w=590  block_height_w=620  block_width=620  block_height=750
  " s_fir_tready" : Outport  SampleTime=Tclk
  " m_fir_tvalid" : Outport  Port=2  SampleTime=Tclk
  IM.O0 : Outport  Port=3  SampleTime=Tclk
  IM.O1 : Outport  Port=4  SampleTime=Tclk
  IM.O2 : Outport  Port=5  SampleTime=Tclk
  IM.O3 : Outport  Port=6  SampleTime=Tclk
  RE.O0 : Outport  Port=7  SampleTime=Tclk
  RE.O1 : Outport  Port=8  SampleTime=Tclk
  RE.O2 : Outport  Port=9  SampleTime=Tclk
  RE.O3 : Outport  Port=10  SampleTime=Tclk
  wires:
  FIR Compiler 7.2 0/2 -> VO/1
  interpolator_in_tvalid/1 -> FIR Compiler 7.2 3/1, FIR Compiler 7.2 2/1, FIR Compiler 7.2 1/1, FIR Compiler 7.2 0/1
  VO/1 -> " m_fir_tvalid"/1
  FIR Compiler 7.2 0/1 -> s_fir_tready/1
  "interp_tvalid "/1 -> interpolator_in_tvalid/1
  s_fir_tready/1 -> " s_fir_tready"/1
  FIR Compiler 7.2 1/3 -> O1.R/1
  "I.RE "/1 -> interpolator_in.RE/1
  "I.IM "/1 -> interpolator_in.IM/1
  FIR Compiler 7.2 0/4 -> O0.I/1
  FIR Compiler 7.2 1/4 -> O1.I/1
  interpolator_in.RE/1 -> FIR Compiler 7.2 0/2, FIR Compiler 7.2 1/2, FIR Compiler 7.2 3/2, FIR Compiler 7.2 2/2
  interpolator_in.IM/1 -> FIR Compiler 7.2 3/3, FIR Compiler 7.2 2/3, FIR Compiler 7.2 1/3, FIR Compiler 7.2 0/3
  FIR Compiler 7.2 3/4 -> O3.I/1
  FIR Compiler 7.2 3/3 -> O3.R/1
  FIR Compiler 7.2 2/4 -> Delay4/1
  FIR Compiler 7.2 2/3 -> Delay5/1
  O0.R/1 -> RE.O0/1
  O0.I/1 -> IM.O0/1
  O1.R/1 -> RE.O1/1
  O1.I/1 -> IM.O1/1
  O2.I/1 -> IM.O2/1
  O2.R/1 -> RE.O2/1
  O3.I/1 -> IM.O3/1
  O3.R/1 -> RE.O3/1
  FIR Compiler 7.2 1/1 -> Terminator1/1
  FIR Compiler 7.2 1/2 -> Terminator2/1
  FIR Compiler 7.2 2/1 -> Terminator3/1
  FIR Compiler 7.2 2/2 -> Terminator/1
  FIR Compiler 7.2 3/1 -> Terminator4/1
  FIR Compiler 7.2 3/2 -> Terminator5/1
  Delay4/1 -> O2.I/1
  Delay5/1 -> O2.R/1
  FIR Compiler 7.2 0/3 -> O0.R/1
